simulink model "C172S_YawDamper_V1"  (R2026a)
settings: Solver=ode4  StartTime=0  StopTime=30  FixedStep=0.01
InitFcn:
  | yd1Data = c172sLateralDirectionalData();
  | [~,yd1Plant] = c172sLateralDirectionalPlant(yd1Data);
  | yd1Controller = c172sYawDamperData();
  | if ~strcmp(yd1Data.model.version,yd1Controller.requiredPlantVersion), error('Yaw Damper plant dependency mismatch.'); end
  | if ~strcmp(yd1Controller.artifactRevision,'YD-V1-MATLAB-R2'), error('Yaw Damper artifact revision mismatch.'); end
  | A_yd1 = yd1Plant.A; B_yd1 = yd1Plant.B;
  | C_yd1 = yd1Plant.C; D_yd1 = yd1Plant.D;
  | Kr_yd1 = yd1Controller.rudderGain_s;
  | Tw_yd1 = yd1Controller.washoutTimeConstant_s;
  | if ~exist('deltaACommand_yd1_rad','var'), deltaACommand_yd1_rad = deg2rad(1.0); end
  | if ~exist('deltaRCommand_yd1_rad','var'), deltaRCommand_yd1_rad = deg2rad(1.0); end
  | if ~exist('x0_yd1','var'), x0_yd1 = zeros(5,1); end
  | if ~exist('xw0_yd1','var'), xw0_yd1 = 0.0; end
undefined symbols (not defined in the file or in its folder): deltaACommand_yd1_rad, deltaRCommand_yd1_rad, x0_yd1, xw0_yd1
settings Model: Creator=Shahi  LastModifiedBy=Shahi

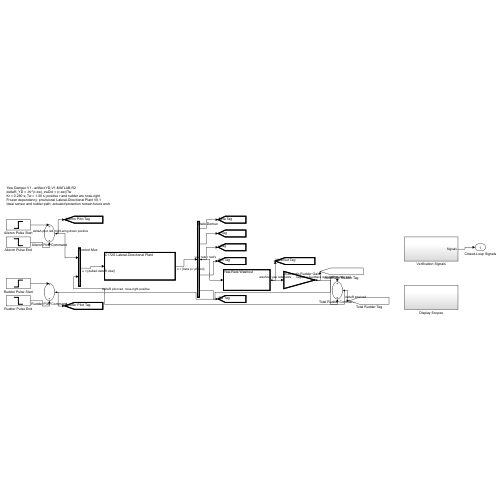
[thumbnail: Simulink's stored preview of the top-level diagram]
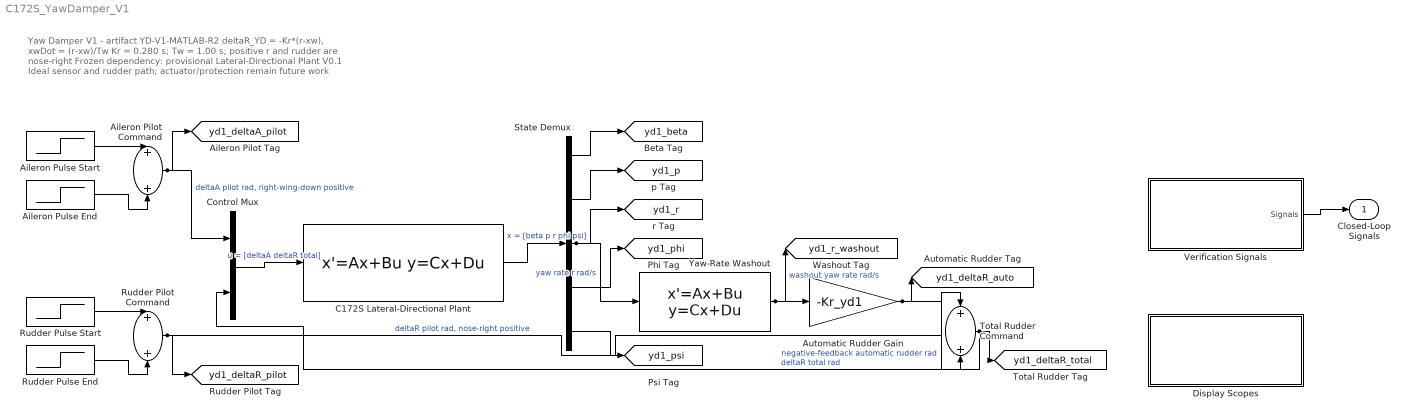
== system C172S_YawDamper_V1 ==
  note: Yaw Damper V1 - artifact YD-V1-MATLAB-R2
      | deltaR_YD = -Kr*(r-xw), xwDot = (r-xw)/Tw
      | Kr = 0.280 s; Tw = 1.00 s; positive r and rudder are nose-right
      | Frozen dependency: provisional Lateral-Directional Plant V0.1
      | Ideal sensor and rudder path; actuator/protection remain future work
  Aileron Pilot Command : Sum
  Aileron Pulse End : Step  FinalValue=-deltaACommand_yd1_rad  SampleTime=0
  Aileron Pulse Start : Step  Time=0  FinalValue=deltaACommand_yd1_rad  SampleTime=0
  Automatic Rudder Gain : Gain  Gain=-Kr_yd1
  C172S Lateral-Directional Plant : StateSpace  A=A_yd1  B=B_yd1  C=C_yd1  D=D_yd1  InitialCondition=x0_yd1
  Control Mux : Mux  Inputs=2
  Display Scopes : Subsystem
  Rudder Pilot Command : Sum
  Rudder Pulse End : Step  Time=6  FinalValue=-deltaRCommand_yd1_rad  SampleTime=0
  Rudder Pulse Start : Step  Time=5  FinalValue=deltaRCommand_yd1_rad  SampleTime=0
  State Demux : Demux  Outputs=5
  Total Rudder Command : Sum
  Verification Signals : Subsystem
  Yaw-Rate Washout : StateSpace  A=-1/Tw_yd1  B=1/Tw_yd1  C=-1  InitialCondition=xw0_yd1
  Closed-Loop Signals : Outport
  tag scope: yd1_beta=global, yd1_deltaA_pilot=global, yd1_deltaR_auto=global, yd1_deltaR_pilot=global, yd1_deltaR_total=global, yd1_p=global, yd1_phi=global, yd1_psi=global, yd1_r=global, yd1_r_washout=global
  wires:
  Verification Signals/1(Signals) -> Closed-Loop Signals/1
  Aileron Pulse Start/1 -> Aileron Pilot Command/1
  Aileron Pulse End/1 -> Aileron Pilot Command/2
  Rudder Pulse Start/1 -> Rudder Pilot Command/1
  Rudder Pulse End/1 -> Rudder Pilot Command/2
  Aileron Pilot Command/1 -> Control Mux/1, [yd1_deltaA_pilot]  "deltaA pilot rad, right-wing-down positive"
  Rudder Pilot Command/1 -> Total Rudder Command/1, [yd1_deltaR_pilot]  "deltaR pilot rad, nose-right positive"
  Total Rudder Command/1 -> Control Mux/2, [yd1_deltaR_total]  "deltaR total rad"
  Control Mux/1 -> C172S Lateral-Directional Plant/1  "u = [deltaA deltaR total]"
  C172S Lateral-Directional Plant/1 -> State Demux/1  "x = [beta p r phi psi]"
  State Demux/3 -> Yaw-Rate Washout/1, [yd1_r]  "yaw rate r rad/s"
  Yaw-Rate Washout/1 -> Automatic Rudder Gain/1, [yd1_r_washout]  "washout yaw rate rad/s"
  Automatic Rudder Gain/1 -> Total Rudder Command/2, [yd1_deltaR_auto]  "negative-feedback automatic rudder rad"
  State Demux/1 -> [yd1_beta]
  State Demux/2 -> [yd1_p]
  State Demux/4 -> [yd1_phi]
  State Demux/5 -> [yd1_psi]

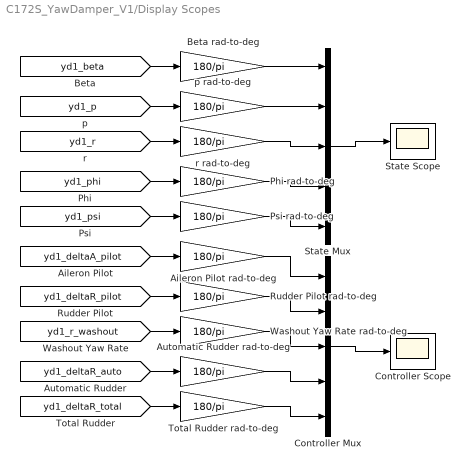
== system C172S_YawDamper_V1/Display Scopes ==
  Aileron Pilot rad-to-deg : Gain  Gain=180/pi
  Automatic Rudder rad-to-deg : Gain  Gain=180/pi
  Beta rad-to-deg : Gain  Gain=180/pi
  Controller Mux : Mux  Inputs=5
  Controller Scope : Scope
  Phi rad-to-deg : Gain  Gain=180/pi
  Psi rad-to-deg : Gain  Gain=180/pi
  Rudder Pilot rad-to-deg : Gain  Gain=180/pi
  State Mux : Mux  Inputs=5
  State Scope : Scope
  Total Rudder rad-to-deg : Gain  Gain=180/pi
  Washout Yaw Rate rad-to-deg : Gain  Gain=180/pi
  p rad-to-deg : Gain  Gain=180/pi
  r rad-to-deg : Gain  Gain=180/pi
  wires:
  [yd1_beta] -> Beta rad-to-deg/1
  [yd1_p] -> p rad-to-deg/1
  [yd1_r] -> r rad-to-deg/1
  [yd1_phi] -> Phi rad-to-deg/1
  [yd1_psi] -> Psi rad-to-deg/1
  [yd1_deltaA_pilot] -> Aileron Pilot rad-to-deg/1
  [yd1_deltaR_pilot] -> Rudder Pilot rad-to-deg/1
  [yd1_r_washout] -> Washout Yaw Rate rad-to-deg/1
  [yd1_deltaR_auto] -> Automatic Rudder rad-to-deg/1
  [yd1_deltaR_total] -> Total Rudder rad-to-deg/1
  Beta rad-to-deg/1 -> State Mux/1
  p rad-to-deg/1 -> State Mux/2
  r rad-to-deg/1 -> State Mux/3
  Phi rad-to-deg/1 -> State Mux/4
  Psi rad-to-deg/1 -> State Mux/5
  State Mux/1 -> State Scope/1
  Aileron Pilot rad-to-deg/1 -> Controller Mux/1
  Rudder Pilot rad-to-deg/1 -> Controller Mux/2
  Washout Yaw Rate rad-to-deg/1 -> Controller Mux/3
  Automatic Rudder rad-to-deg/1 -> Controller Mux/4
  Total Rudder rad-to-deg/1 -> Controller Mux/5
  Controller Mux/1 -> Controller Scope/1

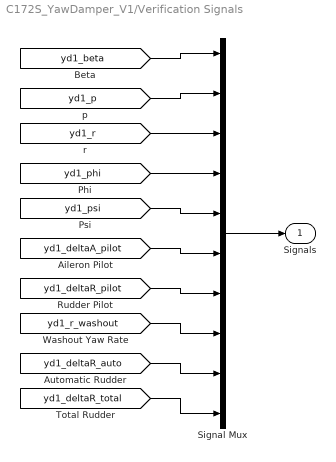
== system C172S_YawDamper_V1/Verification Signals ==
  Signal Mux : Mux  Inputs=10
  Signals : Outport
  wires:
  [yd1_beta] -> Signal Mux/1
  [yd1_p] -> Signal Mux/2
  [yd1_r] -> Signal Mux/3
  [yd1_phi] -> Signal Mux/4
  [yd1_psi] -> Signal Mux/5
  [yd1_deltaA_pilot] -> Signal Mux/6
  [yd1_deltaR_pilot] -> Signal Mux/7
  [yd1_r_washout] -> Signal Mux/8
  [yd1_deltaR_auto] -> Signal Mux/9
  [yd1_deltaR_total] -> Signal Mux/10
  Signal Mux/1 -> Signals/1
